simulink model "montage3"  (Simulink 7.5)
settings: Solver=ode45  StartTime=0.0  StopTime=Tsim  RelTol=1e-3
values from neighbouring files (symbols this model uses):
  Te = 1/Fe    (= 3.125e-06)    [Bode_partie1.m]    (also in fft_script.m = 0.03125; script.m = 0.03125; script1.m; script2.m)
settings Model: Creator=abdala  LastModifiedBy=Yann
settings DebuggingCC: FcnCallInpInsideContextMsg=Enable All
settings GRTTargetCC: CombineOutputUpdateFcns=on

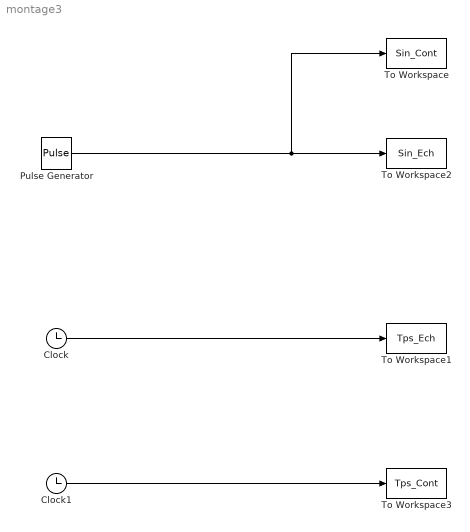
== system montage3 ==
  Clock : Clock
      settings: Decimation=100
  Clock1 : Clock
      settings: Decimation=10
  Pulse Generator : DiscretePulseGenerator  PulseType=Time based  Amplitude=1  Period=1/(85*10^(3))  PulseWidth=50  PhaseDelay=0  SampleTime=1
  To Workspace : ToWorkspace  VariableName=Sin_Cont  SampleTime=Te/100  SaveFormat=Array
  To Workspace1 : ToWorkspace  VariableName=Tps_Ech  SampleTime=Te  SaveFormat=Array
  To Workspace2 : ToWorkspace  VariableName=Sin_Ech  SampleTime=Te  SaveFormat=Array
  To Workspace3 : ToWorkspace  VariableName=Tps_Cont  SampleTime=Te/100  SaveFormat=Array
  wires:
  Pulse Generator/1 -> To Workspace2/1, To Workspace/1
  Clock1/1 -> To Workspace3/1
  Clock/1 -> To Workspace1/1
